simulink model "UAM_Flight_control"  (R2024b)
settings: Solver=FixedStepAuto  StartTime=0.0  StopTime=inf  RelTol=1e-3  EnableMultiTasking=on
undefined symbols (not defined in the file): CityMission, control, controlParams, ControlSampleTime, Cruise_a, DiscIntNeverNeededParam, Earth, FixedWingMission, flightState, FSState, FWControlParams, FWTrimSpeed, HoverMission, params, position, R_WAYPOINTTRANSITION, TransitionMission, uavParam, Vt, w_trim, WGS84, zGround
libraries: slpidlib x56, simulink x32, uavalgslib x7, robotcorelib x2, simulink_extras x2, mspfiltlib x1, aerolibtransform2 x1
(part 12 of 13)

== matlab function UAM_Flight_control/Sensor/Subsystem1/EKF2_Core/EKF2_Algorithm ==
  data: acc input; pos_out output; gyro input; gps_lat input; gps_lon input; gps_alt input; gps_vel input; gps_valid input; baro_alt input; baro_valid input; mag input; mag_valid input; dt input; ref_lat input; ref_lon input; ref_alt input; vel_out output; quat_out output; gyro_bias_out output; accel_bias_out output; wind_vel_out output; terrain_out output; pos_var_out output; vel_var_out output; P_out output; baro_bias_out output; status_out output
function [pos_out, vel_out, quat_out, gyro_bias_out, accel_bias_out, ...
          wind_vel_out, terrain_out, ...
          pos_var_out, vel_var_out, P_out, baro_bias_out, status_out] = ...
    EKF_PX4(acc, gyro, ...
            gps_lat, gps_lon, gps_alt, gps_vel, gps_valid, ...
            baro_alt, baro_valid, ...
            mag, mag_valid, ...
            dt, ref_lat, ref_lon, ref_alt)
%EKF_PX4  PX4 EKF2-equivalent 24-state Extended Kalman Filter (v3.3)
%
%  State vector (24 states):
%    [1:3]   attitude error (rad)      [4:6]   velocity NED (m/s)
%    [7:9]   position NED (m)          [10:12]  gyro bias (rad/s)
%    [13:15] accel bias (m/s^2)        [16:18]  earth mag field (Gauss)
%    [19:21] body mag bias (Gauss)     [22:23]  wind vel NE (m/s)
%    [24]    terrain height (m)
%
%  Update loop (per timestep):
%    1. Buffer sensors  -->  2. Predict state/cov  -->  3. Fuse sensors
%    4. ZUPT / ground damping  -->  5. GSF yaw  -->  6. State resets
%    7. Covariance constraints  -->  8. Output predictor
%
%  Sensors fused:  IMU, GPS (pos/vel/alt), Baro, Magnetometer
%  Not included:   Optical flow, Rangefinder, Airspeed, External vision

% =========================================================================
%  1. TUNING PARAMETERS
% =========================================================================

% --- IMU noise ---
P_GYR_NOISE       = 0.015;       % gyro white noise          (rad/s)
P_ACC_NOISE       = 0.35;        % accel white noise         (m/s^2)
P_GYR_BIAS_NOISE  = 0.001;       % gyro bias random walk     (rad/s^2)
P_ACC_BIAS_NOISE  = 0.01;        % accel bias random walk    (m/s^3)
P_BADACC_PNOISE   = 4.9;         % accel noise during fault  (m/s^2)

% --- Sensor noise ---
P_BARO_NOISE      = 2.0;         % barometer                 (m)
P_GPS_POS_NOISE   = 0.5;         % GPS horizontal position   (m)
P_GPS_VEL_NOISE   = 0.3;         % GPS velocity              (m/s)
P_MAG_NOISE       = 0.05;        % magnetometer body         (Gauss)
P_MAG_BIAS_NOISE  = 0.0001;      % mag body bias drift       (Gauss/s)
P_MAG_EARTH_NOISE = 0.001;       % mag earth field drift     (Gauss/s)
P_HDG_NOISE       = 0.3;         % heading-only mag          (rad)

% --- Environment noise ---
P_WIND_NSD        = 0.1;         % wind velocity             (m/s/sqrt(s))
P_TERR_NOISE      = 5.0;         % terrain height            (m/s)
P_TERR_GRAD       = 0.5;         % terrain gradient          (m/m)

% --- Innovation gates (sigma multiplier) ---
GATE_BARO         = 5.0;
GATE_GPS          = 5.0;
GATE_MAG          = 3.0;
GATE_HDG          = 2.6;

% --- State limits ---
LIM_GYRO_BIAS     = 0.4;         % rad/s
LIM_ACCEL_BIAS    = 0.4;         % m/s^2
LIM_MAG_BIAS      = 0.5;         % Gauss

% --- Bias observability thresholds ---
P_ABL_ACCLIM      = 25.0;        % max accel for bias learn  (m/s^2)
P_ABL_GYRLIM      = 3.0;         % max gyro for bias learn   (rad/s)
P_ABL_TAU         = 0.5;         % maneuver filter tau       (s)
P_IMU_CLIP_THRESH = 39.0;        % IMU clipping threshold    (m/s^2)

% --- Aiding loss fallback ---
P_ZUPT_NOISE      = 0.1;         % zero velocity update      (m/s)
P_ZERO_GYRO_NOISE = 0.01;        % zero gyro update          (rad/s)
P_FAKE_POS_NOISE  = 25.0;        % fake horizontal position  (m)
P_FAKE_HGT_NOISE  = 25.0;        % fake height               (m)

% --- Delay compensation ---
P_GPS_DELAY       = 0.11;        % GPS measurement delay     (s)
BUF_LEN           = 50;          % ring buffer max length

% --- Ground effect ---
P_GND_EFF_DZ      = 4.0;         % propwash deadzone         (m)

% --- EKF-GSF ---
N_GSF             = 5;           % number of GSF models
GSF_RESET_THRESH  = 0.15;        % yaw variance threshold    (rad^2)

% --- Physical constants ---
GRAVITY           = 9.80665;
EARTH_RADIUS      = 6378137.0;
WGS84_E2          = 0.00669437999014;
EARTH_RATE        = 7.2921e-5;    % rad/s

% =========================================================================
%  2. STATE INDICES
% =========================================================================
N_STATES = 24;

IX_ATT = 1:3;       % attitude error
IX_VEL = 4:6;       % velocity NED
IX_POS = 7:9;       % position NED
IX_GB  = 10:12;      % gyro bias
IX_AB  = 13:15;      % accel bias
IX_MI  = 16:18;      % earth magnetic field
IX_MB  = 19:21;      % body magnetic bias
IX_WV  = 22:23;      % wind velocity NE
IX_TR  = 24;         % terrain height

% =========================================================================
%  3. PERSISTENT STATE
% =========================================================================

% --- Core EKF ---
persistent initialized
persistent q_att v_ned p_ned gyro_bias_est accel_bias_est
persistent wind_est terrain_est
persistent P_cov
persistent mag_earth mag_body_bias
persistent baro_bias_est baro_bias_var

% --- Delay ring buffers ---
persistent buf_imu_acc buf_imu_gyro buf_imu_dt
persistent buf_gps_pos buf_gps_vel buf_gps_valid
persistent buf_baro_alt buf_baro_valid
persistent buf_mag_data buf_mag_valid
persistent buf_count delay_steps

% --- Health monitors ---
persistent filt_accel_mag filt_gyro_mag
persistent flag_bad_acc_vert tmr_bad_acc
persistent flag_at_rest tmr_rest
persistent flag_on_ground filt_vibration
persistent lpf_signed_inn tmr_pos_inn tmr_neg_inn
persistent tmr_no_hor_aid tmr_no_ver_aid

% --- Innovation monitors ---
persistent filt_gps_pos_inn filt_gps_vel_inn
persistent tmr_gps_pos_fail tmr_gps_vel_fail
persistent filt_mag_inn tmr_mag_fail

% --- EKF-GSF yaw estimator ---
persistent gsf_yaw gsf_vel gsf_P gsf_weight gsf_converged

% --- Mode flags ---
persistent flag_yaw_aligned flag_mag_3d
persistent cnt_yaw_reset cnt_pos_reset

% --- Output predictor ---
persistent out_q out_v out_p out_initialized

% --- GPS height bias ---
persistent gps_hgt_bias_est gps_hgt_bias_var

% =========================================================================
%  4. INITIALIZATION
% =========================================================================
if isempty(initialized)
    initialized       = false;
    q_att             = [1; 0; 0; 0];
    v_ned             = zeros(3, 1);
    p_ned             = zeros(3, 1);
    gyro_bias_est     = zeros(3, 1);
    accel_bias_est    = zeros(3, 1);
    wind_est          = zeros(2, 1);
    terrain_est       = 0;

    P_cov = diag([ ...
        0.25, 0.25, 0.25, ...       % attitude
        1, 1, 1, ...                 % velocity
        1, 1, 1, ...                 % position
        1e-4, 1e-4, 1e-4, ...       % gyro bias
        0.01, 0.01, 0.01, ...       % accel bias
        0.04, 0.04, 0.04, ...       % mag earth
        0.04, 0.04, 0.04, ...       % mag body
        4, 4, ...                    % wind
        100]);                       % terrain

    mag_earth         = [0.2; 0; 0.4];
    mag_body_bias     = zeros(3, 1);
    baro_bias_est     = 0;
    baro_bias_var     = 1.0;
    gps_hgt_bias_est  = 0;
    gps_hgt_bias_var  = 10.0;

    % Buffers
    buf_imu_acc   = zeros(3, BUF_LEN);
    buf_imu_gyro  = zeros(3, BUF_LEN);
    buf_imu_dt    = zeros(1, BUF_LEN);
    buf_gps_pos   = zeros(3, BUF_LEN);
    buf_gps_vel   = zeros(3, BUF_LEN);
    buf_gps_valid = zeros(1, BUF_LEN);
    buf_baro_alt  = zeros(1, BUF_LEN);
    buf_baro_valid= zeros(1, BUF_LEN);
    buf_mag_data  = zeros(3, BUF_LEN);
    buf_mag_valid = zeros(1, BUF_LEN);
    buf_count     = 0;
    delay_steps   = 0;

    % Monitors
    filt_accel_mag    = GRAVITY;
    filt_gyro_mag     = 0;
    flag_bad_acc_vert = false;
    tmr_bad_acc       = 0;
    flag_at_rest      = true;
    tmr_rest          = 0;
    flag_on_ground    = true;
    filt_vibration    = 0;
    lpf_signed_inn    = 0;
    tmr_pos_inn       = 0;
    tmr_neg_inn       = 0;
    tmr_no_hor_aid    = 0;
    tmr_no_ver_aid    = 0;

    filt_gps_pos_inn  = zeros(2, 1);
    filt_gps_vel_inn  = zeros(3, 1);
    tmr_gps_pos_fail  = 0;
    tmr_gps_vel_fail  = 0;
    filt_mag_inn      = zeros(3, 1);
    tmr_mag_fail      = 0;

    % GSF
    gsf_yaw           = zeros(1, N_GSF);
    gsf_vel           = zeros(2, N_GSF);
    gsf_P             = zeros(3, 3, N_GSF);
    gsf_weight        = ones(1, N_GSF) / N_GSF;
    gsf_converged     = false;

    % Mode
    flag_yaw_aligned  = false;
    flag_mag_3d       = true;
    cnt_yaw_reset     = 0;
    cnt_pos_reset     = 0;

    % Output predictor
    out_q = [1;0;0;0];  out_v = zeros(3,1);  out_p = zeros(3,1);
    out_initialized = false;
end

% =========================================================================
%  5. AUTO-INIT (first valid sensor data)
% =========================================================================
if ~initialized
    delay_steps = min(max(round(P_GPS_DELAY / dt), 1), BUF_LEN);

    % Tilt from accelerometer
    a_norm = acc / max(norm(acc), 1e-6);
    roll0  = atan2(-a_norm(2), -a_norm(3));
    pitch0 = asin(clamp(a_norm(1), -1, 1));

    % Yaw from magnetometer
    yaw0 = 0;
    if mag_valid
        cr = cos(roll0);  sr = sin(roll0);
        cp = cos(pitch0); sp = sin(pitch0);
        mx = mag(1)*cp + mag(2)*sp*sr + mag(3)*sp*cr;
        my = mag(2)*cr - mag(3)*sr;
        yaw0 = atan2(-my, mx);
        flag_yaw_aligned = true;
    end
    q_att = euler2quat(roll0, pitch0, yaw0);

    % Earth magnetic field from first measurement
    if mag_valid
        mag_earth     = quat2dcm(q_att) * mag(:);
        mag_body_bias = zeros(3, 1);
    end

    % Position/velocity from GPS
    if gps_valid
        lat_r = ref_lat * pi / 180;
        p_ned = [(gps_lat - ref_lat) * pi/180 * EARTH_RADIUS;
                 (gps_lon - ref_lon) * pi/180 * EARTH_RADIUS * cos(lat_r);
                 -(gps_alt - ref_alt)];
        v_ned = gps_vel;
    end

    % GSF: spread yaw hypotheses evenly around circle
    for m = 1:N_GSF
        gsf_yaw(m)    = -pi + (m-1) * 2*pi / N_GSF;
        gsf_vel(:, m) = v_ned(1:2);
        gsf_P(:,:,m)  = diag([1, 1, 0.1]);
    end

    out_q = q_att;  out_v = v_ned;  out_p = p_ned;
    initialized = true;
end

% =========================================================================
%  6. SENSOR DELAY BUFFER
% =========================================================================
lat_rad = ref_lat * pi / 180;
gps_ned = [(gps_lat - ref_lat) * pi/180 * EARTH_RADIUS;
           (gps_lon - ref_lon) * pi/180 * EARTH_RADIUS * cos(lat_rad);
           -(gps_alt - ref_alt)];

[d_acc, d_gyro, d_dt, d_gps_ned, d_gps_vel, d_gps_v, ...
 d_baro, d_baro_v, d_mag, d_mag_v] = ...
    push_delay_buffer( ...
        acc, gyro, dt, gps_ned, gps_vel, gps_valid, ...
        baro_alt, baro_valid, mag, mag_valid, ...
        buf_imu_acc, buf_imu_gyro, buf_imu_dt, ...
        buf_gps_pos, buf_gps_vel, buf_gps_valid, ...
        buf_baro_alt, buf_baro_valid, buf_mag_data, buf_mag_valid, ...
        buf_count, delay_steps);

if buf_count < delay_steps
    buf_count = buf_count + 1;
    idx = buf_count;
    buf_imu_acc(:,idx)  = acc;       buf_imu_gyro(:,idx) = gyro;
    buf_imu_dt(idx)     = dt;        buf_gps_pos(:,idx)  = gps_ned;
    buf_gps_vel(:,idx)  = gps_vel;   buf_gps_valid(idx)  = gps_valid;
    buf_baro_alt(idx)   = baro_alt;  buf_baro_valid(idx) = baro_valid;
    buf_mag_data(:,idx) = mag;       buf_mag_valid(idx)  = mag_valid;
else
    % Shift buffers left, push new data to end
    buf_imu_acc  = [buf_imu_acc(:,2:end),  acc];
    buf_imu_gyro = [buf_imu_gyro(:,2:end), gyro];
    buf_imu_dt   = [buf_imu_dt(2:end),     dt];
    buf_gps_pos  = [buf_gps_pos(:,2:end),  gps_ned];
    buf_gps_vel  = [buf_gps_vel(:,2:end),  gps_vel];
    buf_gps_valid= [buf_gps_valid(2:end),  gps_valid];
    buf_baro_alt = [buf_baro_alt(2:end),   baro_alt];
    buf_baro_valid=[buf_baro_valid(2:end),  baro_valid];
    buf_mag_data = [buf_mag_data(:,2:end), mag];
    buf_mag_valid= [buf_mag_valid(2:end),  mag_valid];
end

% =========================================================================
%  7. IMU PREPROCESSING
% =========================================================================
gyro_corrected = d_gyro - gyro_bias_est;
acc_corrected  = d_acc  - accel_bias_est;
imu_clipping   = abs(d_acc) > P_IMU_CLIP_THRESH;

% Filtered maneuver level
alpha_filt = clamp(d_dt / P_ABL_TAU, 0, 1);
filt_accel_mag = max(norm(acc_corrected), (1 - alpha_filt) * filt_accel_mag);
filt_gyro_mag  = max(norm(gyro_corrected),(1 - alpha_filt) * filt_gyro_mag);
is_high_maneuver = (filt_gyro_mag > P_ABL_GYRLIM) || ...
                   (filt_accel_mag > P_ABL_ACCLIM);

% =========================================================================
%  8. FAULT DETECTION
% =========================================================================

% --- Bad vertical accelerometer ---
vert_accel_err = abs(acc_corrected(3) + GRAVITY);
if vert_accel_err > 2.0
    tmr_bad_acc = tmr_bad_acc + d_dt;
    if tmr_bad_acc > 1.0, flag_bad_acc_vert = true; end
else
    tmr_bad_acc = max(tmr_bad_acc - d_dt, 0);
    if tmr_bad_acc < 0.5, flag_bad_acc_vert = false; end
end

% --- Vehicle at rest (requires no vibration) ---
is_gyro_still  = norm(gyro_corrected) < 0.05;
is_accel_still = abs(norm(acc_corrected) - GRAVITY) < 0.5;
is_vel_low     = norm(v_ned) < 0.1;
if is_gyro_still && is_accel_still && is_vel_low
    tmr_rest = tmr_rest + d_dt;
    if tmr_rest > 1.0, flag_at_rest = true; end
else
    tmr_rest = 0;
    flag_at_rest = false;
end

% --- On-ground (works even with motor vibration) ---
is_alt_low = -p_ned(3) < 2.0;
is_vz_low  = abs(v_ned(3)) < 0.5;
flag_on_ground = is_alt_low && (norm(v_ned) < 1.0) && is_vz_low;

% --- Motor vibration detection (proxy for motors active) ---
vib_alpha = clamp(d_dt / 0.5, 0, 1);
filt_vibration = (1 - vib_alpha) * filt_vibration + ...
                  vib_alpha * abs(norm(d_acc) - GRAVITY);
flag_motor_vibration = (filt_vibration > 0.5) && (filt_vibration < 15.0);
flag_gnd_effect = flag_on_ground || (is_alt_low && flag_motor_vibration);

% =========================================================================
%  9. STATE PREDICTION
% =========================================================================

% --- Attitude (exponential map quaternion integration) ---
R_body2ned = quat2dcm(q_att);
earth_rate_NED  = [EARTH_RATE*cos(lat_rad); 0; -EARTH_RATE*sin(lat_rad)];
earth_rate_body = R_body2ned' * earth_rate_NED;

delta_angle = (gyro_corrected - earth_rate_body) * d_dt;
q_pred = qmult(q_att, expmap_quat(delta_angle));
q_pred = q_pred / norm(q_pred);

% --- Velocity (NED frame with Coriolis + transport rate) ---
R_pred = quat2dcm(q_pred);
acc_ned = R_pred * acc_corrected;
coriolis = -2 * cross3(earth_rate_NED, v_ned);

% WGS84 ellipsoid radii of curvature
sin_lat = sin(lat_rad);
den_lat = sqrt(1 - WGS84_E2 * sin_lat^2);
r_meridian = EARTH_RADIUS * (1 - WGS84_E2) / (den_lat^3);
r_prime    = EARTH_RADIUS / den_lat;
altitude   = -p_ned(3);

omega_transport = [ v_ned(2) / (r_prime + altitude);
                   -v_ned(1) / (r_meridian + altitude);
                   -v_ned(2) * tan(lat_rad) / (r_prime + altitude)];
transport = -cross3(omega_transport, v_ned);

v_pred = v_ned + (acc_ned + [0;0;GRAVITY] + coriolis + transport) * d_dt;

% --- Position (trapezoidal integration) ---
p_pred = p_ned + (v_ned + v_pred) * 0.5 * d_dt;

% =========================================================================
%  10. COVARIANCE PREDICTION
% =========================================================================

% State transition Jacobian (first-order)
F = eye(N_STATES);
F(IX_ATT, IX_GB)  = -eye(3) * d_dt;
F(IX_VEL, IX_ATT) = -R_pred * skew3(acc_corrected) * d_dt;
F(IX_VEL, IX_AB)  = -R_pred * d_dt;
F(IX_POS, IX_VEL) =  eye(3) * d_dt;

% Process noise
Q = zeros(N_STATES);
Q(IX_ATT, IX_ATT) = eye(3) * (P_GYR_NOISE * d_dt)^2;
Q(IX_VEL, IX_VEL) = eye(3) * (P_ACC_NOISE * d_dt)^2;

P_pred = F * P_cov * F' + Q;

% Bias process noise (conditional for accel bias)
accel_var = P_ACC_NOISE^2 * ones(3, 1);
if flag_bad_acc_vert || any(imu_clipping)
    accel_var = P_BADACC_PNOISE^2 * ones(3, 1);
end
for i = 1:3
    P_pred(IX_GB(i), IX_GB(i)) = P_pred(IX_GB(i), IX_GB(i)) + ...
                                  (P_GYR_BIAS_NOISE * d_dt)^2;
    if P_pred(IX_AB(i), IX_AB(i)) < accel_var(i)
        P_pred(IX_AB(i), IX_AB(i)) = P_pred(IX_AB(i), IX_AB(i)) + ...
                                      (P_ACC_BIAS_NOISE * d_dt)^2;
    end
end
for i = IX_MI, P_pred(i,i) = P_pred(i,i) + (P_MAG_EARTH_NOISE*d_dt)^2; end
for i = IX_MB, P_pred(i,i) = P_pred(i,i) + (P_MAG_BIAS_NOISE*d_dt)^2;  end
for i = IX_WV, P_pred(i,i) = P_pred(i,i) + (P_WIND_NSD*d_dt)^2;        end

terr_pn = (P_TERR_NOISE*d_dt)^2 + ...
          (P_TERR_GRAD*d_dt)^2 * (v_pred(1)^2 + v_pred(2)^2);
P_pred(IX_TR, IX_TR) = P_pred(IX_TR, IX_TR) + terr_pn;
P_pred = 0.5 * (P_pred + P_pred');

% =========================================================================
%  11. BIAS INHIBIT
% =========================================================================
gb_inhibit = false(3, 1);
ab_inhibit = false(3, 1);
for i = 1:3
    if abs(gyro_corrected(i)) > 5.0
        gb_inhibit(i) = true;
    end
end
inhibit_all_ab = is_high_maneuver || flag_bad_acc_vert;
for i = 1:3
    ab_inhibit(i) = inhibit_all_ab || imu_clipping(i);
    if ~flag_at_rest && abs(R_pred(3,i)) < sin(15*pi/180)
        ab_inhibit(i) = true;        % not observable
    end
end

% =========================================================================
%  12. MEASUREMENT UPDATES (sequential scalar fusion)
% =========================================================================
q_u  = q_pred;     v_u  = v_pred;    p_u  = p_pred;
gb_u = gyro_bias_est;  ab_u = accel_bias_est;
wv_u = wind_est;   tr_u = terrain_est;
P_u  = P_pred;

did_fuse_gps = false;
did_fuse_hgt = false;
mag_hdg_ratio = 0;

% Shorthand for repeated fusion call arguments
FARGS = {IX_ATT, IX_VEL, IX_POS, IX_GB, IX_AB, ...
         IX_MI, IX_MB, IX_WV, IX_TR, ...
         LIM_GYRO_BIAS, LIM_ACCEL_BIAS, LIM_MAG_BIAS};

% ----- 12a. BAROMETER HEIGHT (primary reference) -----------------------
if d_baro_v
    H_b = zeros(1, N_STATES);  H_b(9) = 1;
    obs_baro = -(d_baro - ref_alt) - baro_bias_est;
    inn_b = obs_baro - p_u(3);

    % One-sided deadzone: suppress only negative innovations (propwash)
    %   inn_b < 0 means baro reads higher than EKF (low pressure from propwash)
    %   If |inn_b| < DZ  → zero out (inside deadzone)
    %   If |inn_b| >= DZ → shift by DZ toward zero
    R_baro = P_BARO_NOISE;
    if flag_gnd_effect && P_GND_EFF_DZ > 0
        if inn_b < 0
            if inn_b > -P_GND_EFF_DZ
                inn_b = 0;                    % inside deadzone
            else
                inn_b = inn_b + P_GND_EFF_DZ; % shift toward zero
            end
        end
        if flag_motor_vibration
            R_baro = P_BARO_NOISE * 3.0;
        end
    end

    S_b = H_b * P_u * H_b' + R_baro^2;
    test_ratio = inn_b^2 / (GATE_BARO^2 * S_b);

    % Clamp during bad vertical accel (don't reject, just limit)
    if flag_bad_acc_vert && test_ratio >= 1.0
        inn_b = clamp(inn_b, -GATE_BARO*sqrt(S_b), GATE_BARO*sqrt(S_b));
        test_ratio = 0.99;
    end

    if test_ratio < 1.0
        K_b = P_u * H_b' / S_b;
        K_b = apply_inhibit(K_b, gb_inhibit, ab_inhibit, IX_GB, IX_AB);
        [q_u,v_u,p_u,gb_u,ab_u,mag_earth,mag_body_bias,wv_u,tr_u] = ...
            fuse_state(q_u,v_u,p_u,gb_u,ab_u,mag_earth,mag_body_bias, ...
                       wv_u,tr_u, K_b, inn_b, FARGS{:});
        P_u = joseph_update(P_u, K_b, H_b, R_baro^2, N_STATES);
        did_fuse_hgt = true;
        tmr_no_ver_aid = 0;
    end
end

% ----- 12b. BARO BIAS ESTIMATOR ----------------------------------------
BIAS_MON_TIME = 10.0;
baro_bias_pn = 0.01^2 * d_dt;
if abs(lpf_signed_inn) > 0.2 || tmr_pos_inn > BIAS_MON_TIME || ...
   tmr_neg_inn > BIAS_MON_TIME
    baro_bias_pn = baro_bias_pn * 10.0;
end
if flag_gnd_effect && flag_motor_vibration
    baro_bias_pn = baro_bias_pn * 50.0;  % fast tracking during propwash
end
baro_bias_var = clamp(baro_bias_var + baro_bias_pn, 1e-8, 100);

if d_baro_v
    bi = (-(d_baro - ref_alt) + p_u(3)) - baro_bias_est;
    Si = baro_bias_var + P_BARO_NOISE^2 + P_u(9,9);
    tr_bi = bi^2 / (25 * Si);
    if tr_bi < 1.0
        Kb = baro_bias_var / Si;
        baro_bias_est = baro_bias_est + Kb * bi;
        baro_bias_var = (1 - Kb) * baro_bias_var;
    end
    lpf_a = clamp(d_dt / BIAS_MON_TIME, 0, 1);
    lpf_signed_inn = (1-lpf_a)*lpf_signed_inn + lpf_a*sign(bi)*min(tr_bi,1);
    if bi > 0
        tmr_pos_inn = 0;  tmr_neg_inn = tmr_neg_inn + d_dt;
    else
        tmr_neg_inn = 0;  tmr_pos_inn = tmr_pos_inn + d_dt;
    end
end

% ----- 12c. GPS HORIZONTAL POSITION ------------------------------------
gps_pos_rejected = false;
if d_gps_v
    rej_cnt = 0;
    for ax = 1:2
        H = zeros(1,N_STATES);  H(6+ax) = 1;
        inn = d_gps_ned(ax) - p_u(ax);
        S = H*P_u*H' + P_GPS_POS_NOISE^2;
        tr = inn^2 / (GATE_GPS^2 * S);

        af = clamp(d_dt / 0.5, 0, 1);
        filt_gps_pos_inn(ax) = (1-af)*filt_gps_pos_inn(ax) + ...
                                af*sign(inn)*min(tr, 1);
        if tr < 1.0
            K = apply_inhibit(P_u*H'/S, gb_inhibit, ab_inhibit, IX_GB, IX_AB);
            [q_u,v_u,p_u,gb_u,ab_u,mag_earth,mag_body_bias,wv_u,tr_u] = ...
                fuse_state(q_u,v_u,p_u,gb_u,ab_u,mag_earth,mag_body_bias,...
                           wv_u,tr_u, K, inn, FARGS{:});
            P_u = joseph_update(P_u, K, H, P_GPS_POS_NOISE^2, N_STATES);
            did_fuse_gps = true;
            tmr_no_hor_aid = 0;
        else
            rej_cnt = rej_cnt + 1;
        end
    end
    gps_pos_rejected = (rej_cnt == 2);
end
tmr_gps_pos_fail = update_fail_timer(tmr_gps_pos_fail, ...
                    gps_pos_rejected || ~d_gps_v, d_dt);

% ----- 12d. GPS VELOCITY -----------------------------------------------
gps_vel_rejected = false;
if d_gps_v
    rej_cnt = 0;
    for ax = 1:3
        H = zeros(1,N_STATES);  H(3+ax) = 1;
        inn = d_gps_vel(ax) - v_u(ax);
        R_v = P_GPS_VEL_NOISE^2;
        if ax == 3, R_v = (1.5 * P_GPS_VEL_NOISE)^2; end  % vz: 1.5x noise
        S = H*P_u*H' + R_v;
        tr = inn^2 / (GATE_GPS^2 * S);

        af = clamp(d_dt / 0.5, 0, 1);
        filt_gps_vel_inn(ax) = (1-af)*filt_gps_vel_inn(ax) + ...
                                af*sign(inn)*min(tr, 1);
        if tr < 1.0
            K = apply_inhibit(P_u*H'/S, gb_inhibit, ab_inhibit, IX_GB, IX_AB);
            [q_u,v_u,p_u,gb_u,ab_u,mag_earth,mag_body_bias,wv_u,tr_u] = ...
                fuse_state(q_u,v_u,p_u,gb_u,ab_u,mag_earth,mag_body_bias,...
                           wv_u,tr_u, K, inn, FARGS{:});
            P_u = joseph_update(P_u, K, H, R_v, N_STATES);
            did_fuse_gps = true;
        else
            rej_cnt = rej_cnt + 1;
        end
    end
    gps_vel_rejected = (rej_cnt == 3);
end
tmr_gps_vel_fail = update_fail_timer(tmr_gps_vel_fail, ...
                    gps_vel_rejected || ~d_gps_v, d_dt);

% ----- 12e. GPS ALTITUDE (with bias estimator) -------------------------
gps_hgt_bias_var = min(gps_hgt_bias_var + 0.02^2 * d_dt, 100);
if d_gps_v
    H = zeros(1,N_STATES);  H(9) = 1;
    R_ga = (1.5 * P_GPS_POS_NOISE)^2;
    obs_gps_z = d_gps_ned(3) - gps_hgt_bias_est;
    inn = obs_gps_z - p_u(3);
    S = H*P_u*H' + R_ga + gps_hgt_bias_var;

    if flag_bad_acc_vert
        inn = clamp(inn, -GATE_GPS*sqrt(S), GATE_GPS*sqrt(S));
    end
    if inn^2 < GATE_GPS^2 * S
        K = apply_inhibit(P_u*H'/S, gb_inhibit, ab_inhibit, IX_GB, IX_AB);
        [q_u,v_u,p_u,gb_u,ab_u,mag_earth,mag_body_bias,wv_u,tr_u] = ...
            fuse_state(q_u,v_u,p_u,gb_u,ab_u,mag_earth,mag_body_bias,...
                       wv_u,tr_u, K, inn, FARGS{:});
        P_u = joseph_update(P_u, K, H, R_ga + gps_hgt_bias_var, N_STATES);
        did_fuse_hgt = true;
        tmr_no_ver_aid = 0;
    end

    % Bias estimator update
    gi = d_gps_ned(3) - p_u(3) - gps_hgt_bias_est;
    Si_g = gps_hgt_bias_var + R_ga + P_u(9,9);
    if gi^2 < 25*Si_g && Si_g > 1e-6
        Kg = gps_hgt_bias_var / Si_g;
        gps_hgt_bias_est = gps_hgt_bias_est + Kg * gi;
        gps_hgt_bias_var = (1 - Kg) * gps_hgt_bias_var;
    end
end

% ----- 12f. MAGNETOMETER -----------------------------------------------
R_dcm = quat2dcm(q_u);
R_dcm_t = R_dcm';
pitch_now = asin(clamp(-R_dcm(1,3), -1, 1));

% Mode selection: 3D or heading-only
mag_disturbed = false;
if d_mag_v
    if abs(norm(d_mag) - norm(mag_earth)) > 0.3 * norm(mag_earth)
        mag_disturbed = true;
    end
end
if abs(pitch_now) > 60*pi/180 || tmr_mag_fail > 3.0 || mag_disturbed
    flag_mag_3d = false;
else
    flag_mag_3d = true;
end

if d_mag_v
    if flag_mag_3d
        % --- 3D magnetometer fusion ---
        mag_pred = R_dcm_t * mag_earth + mag_body_bias;
        allow_tilt = abs(pitch_now) < 45*pi/180;
        mag_rej = 0;

        for ax = 1:3
            dMdA = -R_dcm_t * skew3(mag_earth);
            H = zeros(1,N_STATES);
            H(IX_ATT) = dMdA(ax,:);
            H(IX_MI)  = R_dcm_t(ax,:);
            H(IX_MB(ax)) = 1;

            inn = d_mag(ax) - mag_pred(ax);
            S = H*P_u*H' + P_MAG_NOISE^2;
            tr = inn^2 / (GATE_MAG^2 * S);

            af = clamp(d_dt / 0.5, 0, 1);
            filt_mag_inn(ax) = (1-af)*filt_mag_inn(ax) + af*sign(inn)*min(tr,1);

            if tr < 1.0 && S > 0
                K = apply_inhibit(P_u*H'/S, gb_inhibit, ab_inhibit, IX_GB, IX_AB);
                if ~allow_tilt
                    K(1) = 0;  K(2) = 0;
                    K(IX_GB(1)) = 0;  K(IX_GB(2)) = 0;
                end
                [q_u,v_u,p_u,gb_u,ab_u,mag_earth,mag_body_bias,wv_u,tr_u]=...
                    fuse_state(q_u,v_u,p_u,gb_u,ab_u,mag_earth,...
                               mag_body_bias,wv_u,tr_u,K,inn,FARGS{:});
                P_u = joseph_update(P_u, K, H, P_MAG_NOISE^2, N_STATES);

                R_dcm = quat2dcm(q_u);  R_dcm_t = R_dcm';
                mag_pred = R_dcm_t * mag_earth + mag_body_bias;
            else
                mag_rej = mag_rej + 1;
            end
        end
        tmr_mag_fail = update_fail_timer(tmr_mag_fail, mag_rej==3, d_dt);

    else
        % --- Heading-only magnetometer fusion ---
        mag_NED = R_dcm * d_mag;
        Bx = mag_NED(1);  By = mag_NED(2);
        D_meas = Bx^2 + By^2;
        D_pred = mag_earth(1)^2 + mag_earth(2)^2;

        if D_meas > 0.01 && D_pred > 0.01
            inn = wrapToPi(atan2(By, Bx) - atan2(mag_earth(2), mag_earth(1)));

            H = zeros(1, N_STATES);
            H(3) = -1;                                 % yaw only
            H(IX_MI(1)) =  mag_earth(2) / D_pred;
            H(IX_MI(2)) = -mag_earth(1) / D_pred;

            S = H*P_u*H' + P_HDG_NOISE^2;
            tr = inn^2 / (GATE_HDG^2 * S);
            mag_hdg_ratio = tr;

            if tr < 1.0 && S > 0
                K = apply_inhibit(P_u*H'/S, gb_inhibit, ab_inhibit, IX_GB, IX_AB);
                K(1) = 0;  K(2) = 0;
                K(IX_GB(1)) = 0;  K(IX_GB(2)) = 0;
                [q_u,v_u,p_u,gb_u,ab_u,mag_earth,mag_body_bias,wv_u,tr_u]=...
                    fuse_state(q_u,v_u,p_u,gb_u,ab_u,mag_earth,...
                               mag_body_bias,wv_u,tr_u,K,inn,FARGS{:});
                P_u = joseph_update(P_u, K, H, P_HDG_NOISE^2, N_STATES);
                tmr_mag_fail = max(tmr_mag_fail - d_dt, 0);
            else
                tmr_mag_fail = tmr_mag_fail + d_dt;
            end
        end
    end
end

% ----- 12g. GRAVITY VECTOR FUSION --------------------------------------
if ~is_high_maneuver && ~flag_bad_acc_vert
    acc_mag = norm(acc_corrected);
    if acc_mag > 0.5*GRAVITY && acc_mag < 1.5*GRAVITY
        R_g = quat2dcm(q_u);
        grav_pred = R_g' * [0;0;GRAVITY];
        grav_meas = acc_corrected / acc_mag * GRAVITY;
        R_grav = 1.0;

        for ax = 1:2
            dGdA = -R_g' * skew3([0;0;GRAVITY]);
            H_g = zeros(1, N_STATES);
            H_g(IX_ATT) = dGdA(ax,:);
            H_g(IX_AB(ax)) = -1;

            inn_g = grav_meas(ax) - grav_pred(ax);
            S_g = H_g*P_u*H_g' + R_grav;
            if inn_g^2 < 9*S_g && S_g > 0
                K_g = apply_inhibit(P_u*H_g'/S_g, gb_inhibit, ab_inhibit, IX_GB, IX_AB);
                K_g(3) = 0;  K_g(IX_GB(3)) = 0;    % no yaw from gravity
                [q_u,v_u,p_u,gb_u,ab_u,mag_earth,mag_body_bias,wv_u,tr_u]=...
                    fuse_state(q_u,v_u,p_u,gb_u,ab_u,mag_earth,...
                               mag_body_bias,wv_u,tr_u,K_g,inn_g,FARGS{:});
                P_u = joseph_update(P_u, K_g, H_g, R_grav, N_STATES);
            end
        end
    end
end

% =========================================================================
%  13. VELOCITY CONSTRAINTS
% =========================================================================

% --- ZUPT (vehicle at rest) ---
if flag_at_rest
    for ax = 1:3
        H = zeros(1,N_STATES);  H(3+ax) = 1;
        inn = -v_u(ax);
        S = H*P_u*H' + P_ZUPT_NOISE^2;
        if inn^2 < 25*S
            K = apply_inhibit(P_u*H'/S, gb_inhibit, ab_inhibit, IX_GB, IX_AB);
            [q_u,v_u,p_u,gb_u,ab_u,mag_earth,mag_body_bias,wv_u,tr_u]=...
                fuse_state(q_u,v_u,p_u,gb_u,ab_u,mag_earth,...
                           mag_body_bias,wv_u,tr_u,K,inn,FARGS{:});
            P_u = joseph_update(P_u, K, H, P_ZUPT_NOISE^2, N_STATES);
        end
    end
end

% --- On-ground velocity damping (motors running but not flying) ---
if flag_on_ground && ~flag_at_rest
    % Vertical velocity → zero (tight)
    H = zeros(1,N_STATES);  H(6) = 1;
    inn_vz = -v_u(3);
    R_vz = 0.5^2;
    S_vz = H*P_u*H' + R_vz;
    if inn_vz^2 < 25*S_vz
        K = apply_inhibit(P_u*H'/S_vz, gb_inhibit, ab_inhibit, IX_GB, IX_AB);
        [q_u,v_u,p_u,gb_u,ab_u,mag_earth,mag_body_bias,wv_u,tr_u]=...
            fuse_state(q_u,v_u,p_u,gb_u,ab_u,mag_earth,...
                       mag_body_bias,wv_u,tr_u,K,inn_vz,FARGS{:});
        P_u = joseph_update(P_u, K, H, R_vz, N_STATES);
    end

    % Horizontal velocity → zero (looser)
    R_vh = 2.0^2;
    for ax = 1:2
        H = zeros(1,N_STATES);  H(3+ax) = 1;
        inn_vh = -v_u(ax);
        S_vh = H*P_u*H' + R_vh;
        if inn_vh^2 < 25*S_vh
            K = apply_inhibit(P_u*H'/S_vh, gb_inhibit, ab_inhibit, IX_GB, IX_AB);
            [q_u,v_u,p_u,gb_u,ab_u,mag_earth,mag_body_bias,wv_u,tr_u]=...
                fuse_state(q_u,v_u,p_u,gb_u,ab_u,mag_earth,...
                           mag_body_bias,wv_u,tr_u,K,inn_vh,FARGS{:});
            P_u = joseph_update(P_u, K, H, R_vh, N_STATES);
        end
    end
end

% --- Zero gyro update (at rest only) ---
if flag_at_rest
    for ax = 1:3
        H = zeros(1,N_STATES);  H(IX_GB(ax)) = -1;
        inn = -(d_gyro(ax) - gb_u(ax));
        S = H*P_u*H' + P_ZERO_GYRO_NOISE^2;
        if S > 0 && inn^2 < 25*S
            K = P_u*H'/S;
            [q_u,v_u,p_u,gb_u,ab_u,mag_earth,mag_body_bias,wv_u,tr_u]=...
                fuse_state(q_u,v_u,p_u,gb_u,ab_u,mag_earth,...
                           mag_body_bias,wv_u,tr_u,K,inn,FARGS{:});
            P_u = joseph_update(P_u, K, H, P_ZERO_GYRO_NOISE^2, N_STATES);
        end
    end
end

% --- Fake position / height aiding ---
if ~did_fuse_gps, tmr_no_hor_aid = tmr_no_hor_aid + d_dt; end
if ~did_fuse_hgt, tmr_no_ver_aid = tmr_no_ver_aid + d_dt; end

if tmr_no_hor_aid > 5.0
    for ax = 1:2
        H = zeros(1,N_STATES);  H(6+ax) = 1;
        S = H*P_u*H' + P_FAKE_POS_NOISE^2;
        P_u = joseph_update(P_u, P_u*H'/S, H, P_FAKE_POS_NOISE^2, N_STATES);
    end
end
if tmr_no_ver_aid > 5.0
    H = zeros(1,N_STATES);  H(9) = 1;
    S = H*P_u*H' + P_FAKE_HGT_NOISE^2;
    P_u = joseph_update(P_u, P_u*H'/S, H, P_FAKE_HGT_NOISE^2, N_STATES);
end

% =========================================================================
%  14. EKF-GSF YAW ESTIMATOR
% =========================================================================
[roll_now, pitch_now_e, yaw_now] = quat2euler(q_u);

% Predict all models
for m = 1:N_GSF
    sr = sin(roll_now);  cr = cos(roll_now);  cp = cos(pitch_now_e);
    yaw_rate = gyro_corrected(3);
    if abs(cp) > 1e-6
        yaw_rate = gyro_corrected(2)*sr/cp + gyro_corrected(3)*cr/cp;
    end
    gsf_yaw(m) = wrapToPi(gsf_yaw(m) + yaw_rate * d_dt);

    R_gsf = euler2dcm(roll_now, pitch_now_e, gsf_yaw(m));
    a_ned = R_gsf * acc_corrected;
    gsf_vel(:,m) = gsf_vel(:,m) + a_ned(1:2) * d_dt;

    cy = cos(gsf_yaw(m));  sy = sin(gsf_yaw(m));
    dv_dpsi = [(-acc_corrected(1)*sy - acc_corrected(2)*cy) * d_dt;
               ( acc_corrected(1)*cy - acc_corrected(2)*sy) * d_dt];
    Fm = eye(3);  Fm(1,3) = dv_dpsi(1);  Fm(2,3) = dv_dpsi(2);
    Qm = diag([(P_ACC_NOISE*d_dt)^2, (P_ACC_NOISE*d_dt)^2, (P_GYR_NOISE*d_dt)^2]);
    gsf_P(:,:,m) = Fm * gsf_P(:,:,m) * Fm' + Qm;
end

% Update with GPS velocity
if d_gps_v && did_fuse_gps
    for m = 1:N_GSF
        inn_g = d_gps_vel(1:2) - gsf_vel(:,m);
        cy = cos(gsf_yaw(m));  sy = sin(gsf_yaw(m));
        dv = [(-acc_corrected(1)*sy - acc_corrected(2)*cy)*d_dt;
              ( acc_corrected(1)*cy - acc_corrected(2)*sy)*d_dt];
        Hm = [1,0,dv(1); 0,1,dv(2)];
        Rm = P_GPS_VEL_NOISE^2 * eye(2);
        Sm = Hm * gsf_P(:,:,m) * Hm' + Rm;

        det_S = Sm(1,1)*Sm(2,2) - Sm(1,2)*Sm(2,1);
        if det_S > 1e-6
            Si = [Sm(2,2),-Sm(1,2); -Sm(2,1),Sm(1,1)] / det_S;

            nis = inn_g' * Si * inn_g;
            if nis > 25, inn_g = inn_g * sqrt(25/nis); nis = 25; end

            Km = gsf_P(:,:,m) * Hm' * Si;
            dx = Km * inn_g;
            gsf_vel(:,m) = gsf_vel(:,m) + dx(1:2);
            gsf_yaw(m) = wrapToPi(gsf_yaw(m) + dx(3));
            gsf_P(:,:,m) = (eye(3) - Km*Hm) * gsf_P(:,:,m);

            gsf_weight(m) = gsf_weight(m) * exp(-0.5*nis) / sqrt(abs(det_S));
        end
    end
    wt_sum = sum(gsf_weight);
    if wt_sum > 1e-30
        gsf_weight = gsf_weight / wt_sum;
    else
        gsf_weight = ones(1,N_GSF) / N_GSF;
    end
end

% Composite estimate
s_sum = sum(gsf_weight .* sin(gsf_yaw));
c_sum = sum(gsf_weight .* cos(gsf_yaw));
gsf_yaw_est = atan2(s_sum, c_sum);

% Mixture variance
gsf_yaw_var = 0;
for m = 1:N_GSF
    d_yaw = wrapToPi(gsf_yaw(m) - gsf_yaw_est);
    gsf_yaw_var = gsf_yaw_var + gsf_weight(m) * (gsf_P(3,3,m) + d_yaw^2);
end
gsf_yaw_var = max(gsf_yaw_var, 1e-4);
gsf_converged = gsf_yaw_var < GSF_RESET_THRESH;

% =========================================================================
%  15. STATE RESETS
% =========================================================================

% --- Yaw reset from GSF ---
yaw_failing = tmr_mag_fail > 5.0 || mag_hdg_ratio > 1.0;
if gsf_converged && (~flag_yaw_aligned || (yaw_failing && ~flag_at_rest))
    dq = euler2quat(0, 0, wrapToPi(gsf_yaw_est - yaw_now));
    q_u = qmult(dq, q_u);
    q_u = q_u / norm(q_u);
    P_u(3,:) = 0;  P_u(:,3) = 0;
    P_u(3,3) = max(gsf_yaw_var, 1e-4);
    flag_yaw_aligned = true;
    cnt_yaw_reset = cnt_yaw_reset + 1;
    tmr_mag_fail = 0;
end

% --- Position reset from GPS ---
if tmr_gps_pos_fail > 5.0 && d_gps_v && ~gps_pos_rejected
    p_u(1:2) = d_gps_ned(1:2);
    P_u(7,:)=0; P_u(:,7)=0; P_u(8,:)=0; P_u(:,8)=0;
    P_u(7,7) = P_GPS_POS_NOISE^2;
    P_u(8,8) = P_GPS_POS_NOISE^2;
    tmr_gps_pos_fail = 0;
    cnt_pos_reset = cnt_pos_reset + 1;
end

% --- Velocity reset from GPS ---
if tmr_gps_vel_fail > 5.0 && d_gps_v && ~gps_vel_rejected
    v_u = d_gps_vel;
    for ax = 4:6
        P_u(ax,:)=0; P_u(:,ax)=0;
    end
    P_u(4,4)=P_GPS_VEL_NOISE^2; P_u(5,5)=P_GPS_VEL_NOISE^2;
    P_u(6,6)=P_GPS_VEL_NOISE^2;
    tmr_gps_vel_fail = 0;
end

% =========================================================================
%  16. COVARIANCE HEALTH
% =========================================================================
cov_max = [1,1,1, 1e6,1e6,1e6, 1e6,1e6,1e6, .1,.1,.1, .1,.1,.1, ...
           1,1,1, 1,1,1, 1e6,1e6, 1e4];
cov_min = [1e-9,1e-9,1e-9, 1e-6,1e-6,1e-6, 1e-6,1e-6,1e-6, ...
           1e-9,1e-9,1e-9, 1e-9,1e-9,1e-9, 1e-6,1e-6,1e-6, ...
           1e-6,1e-6,1e-6, 1e-6,1e-6, 0];

for i = 1:N_STATES
    if P_u(i,i) < cov_min(i)
        P_u(i,i) = cov_min(i);
    elseif P_u(i,i) > cov_max(i)
        % Fuse zero-innovation to reduce ~10% (preserves cross-correlation)
        R_s = 10 * P_u(i,i);
        Hs = zeros(1,N_STATES);  Hs(i) = 1;
        P_u = joseph_update(P_u, P_u*Hs'/(P_u(i,i)+R_s), Hs, R_s, N_STATES);
    end
end
P_u = 0.5 * (P_u + P_u');

% =========================================================================
%  17. STORE DELAYED STATE
% =========================================================================
q_att         = q_u;
v_ned         = v_u;
p_ned         = p_u;
gyro_bias_est = gb_u;
accel_bias_est= ab_u;
wind_est      = wv_u;
terrain_est   = tr_u;
P_cov         = P_u;

% =========================================================================
%  18. OUTPUT PREDICTOR (replay IMU from delayed → current time)
% =========================================================================
oq = q_u;  ov = v_u;  op = p_u;

if buf_count >= delay_steps && delay_steps > 0
    for k = 1:delay_steps
        gk = buf_imu_gyro(:,k) - gb_u;
        ak = buf_imu_acc(:,k)  - ab_u;
        dtk = buf_imu_dt(k);

        Rk = quat2dcm(oq);
        d_ang = (gk - Rk' * earth_rate_NED) * dtk;
        oq = qmult(oq, expmap_quat(d_ang));
        oq = oq / norm(oq);

        a_ned_k = quat2dcm(oq) * ak;
        ov = ov + (a_ned_k + [0;0;GRAVITY]) * dtk;
        op = op + ov * dtk;
    end
end

% Smooth transition (prevent output jumps)
TAU_SMOOTH = 0.15;
alpha_s = clamp(dt / (dt + TAU_SMOOTH), 0, 1);

if out_initialized
    out_v = out_v + alpha_s * (ov - out_v);
    out_p = out_p + alpha_s * (op - out_p);

    q_err = qmult(qconj(out_q), oq);
    if q_err(1) < 0, q_err = -q_err; end
    att_corr = alpha_s * 2 * q_err(2:4);
    out_q = qmult(expmap_quat(att_corr), out_q);
    out_q = out_q / norm(out_q);
else
    out_q = oq;  out_v = ov;  out_p = op;
    out_initialized = true;
end

% =========================================================================
%  19. OUTPUTS
% =========================================================================
status_out = [ ...
    double(flag_at_rest);        %  1: vehicle at rest
    double(flag_bad_acc_vert);   %  2: bad vertical accel
    double(tmr_no_hor_aid>10);   %  3: horizontal dead reckoning
    double(tmr_no_ver_aid>10);   %  4: vertical dead reckoning
    double(did_fuse_gps);        %  5: GPS fused this step
    double(did_fuse_hgt);        %  6: height fused this step
    double(flag_yaw_aligned);    %  7: yaw is aligned
    double(gsf_converged);       %  8: GSF yaw converged
    double(flag_mag_3d);         %  9: using 3D mag fusion
    double(cnt_yaw_reset)];      % 10: yaw reset count

quat_out       = out_q;
vel_out        = out_v;
pos_out        = out_p;
gyro_bias_out  = gb_u;
accel_bias_out = ab_u;
wind_vel_out   = wv_u;
terrain_out    = tr_u;
baro_bias_out  = baro_bias_est;
P_out          = P_u;
pos_var_out    = [P_u(7,7); P_u(8,8); P_u(9,9)];
vel_var_out    = [P_u(4,4); P_u(5,5); P_u(6,6)];
end


% #########################################################################
%  HELPER FUNCTIONS
% #########################################################################

% ---- Clamp value to [lo, hi] -------------------------------------------
function y = clamp(x, lo, hi)
    y = min(max(x, lo), hi);
end

% ---- Skew-symmetric matrix ---------------------------------------------
function S = skew3(v)
    S = [0,-v(3),v(2); v(3),0,-v(1); -v(2),v(1),0];
end

% ---- Cross product ------------------------------------------------------
function c = cross3(a, b)
    c = [a(2)*b(3)-a(3)*b(2); a(3)*b(1)-a(1)*b(3); a(1)*b(2)-a(2)*b(1)];
end

% ---- Quaternion → DCM (body-to-NED) ------------------------------------
function R = quat2dcm(q)
    w=q(1); x=q(2); y=q(3); z=q(4);
    R = [w^2+x^2-y^2-z^2,  2*(x*y-w*z),      2*(x*z+w*y);
         2*(x*y+w*z),      w^2-x^2+y^2-z^2,  2*(y*z-w*x);
         2*(x*z-w*y),      2*(y*z+w*x),      w^2-x^2-y^2+z^2];
end

% ---- Euler → DCM -------------------------------------------------------
function R = euler2dcm(r, p, y)
    cr=cos(r); sr=sin(r); cp=cos(p); sp=sin(p); cy=cos(y); sy=sin(y);
    R = [cp*cy,          cp*sy,          -sp;
         sr*sp*cy-cr*sy, sr*sp*sy+cr*cy,  sr*cp;
         cr*sp*cy+sr*sy, cr*sp*sy-sr*cy,  cr*cp];
end

% ---- Euler → Quaternion -------------------------------------------------
function q = euler2quat(r, p, y)
    cr=cos(r/2); sr=sin(r/2);
    cp=cos(p/2); sp=sin(p/2);
    cy=cos(y/2); sy=sin(y/2);
    q = [cr*cp*cy + sr*sp*sy;
         sr*cp*cy - cr*sp*sy;
         cr*sp*cy + sr*cp*sy;
         cr*cp*sy - sr*sp*cy];
end

% ---- Quaternion → Euler -------------------------------------------------
function [r, p, y] = quat2euler(q)
    w=q(1); x=q(2); y_=q(3); z=q(4);
    r = atan2(2*(w*x + y_*z), 1 - 2*(x^2 + y_^2));
    p = asin(max(min(2*(w*y_ - z*x), 1), -1));
    y = atan2(2*(w*z + x*y_), 1 - 2*(y_^2 + z^2));
end

% ---- Quaternion conjugate -----------------------------------------------
function qc = qconj(q)
    qc = [q(1); -q(2); -q(3); -q(4)];
end

% ---- Quaternion multiplication ------------------------------------------
function qo = qmult(a, b)
    qo = [a(1)*b(1)-a(2)*b(2)-a(3)*b(3)-a(4)*b(4);
          a(1)*b(2)+a(2)*b(1)+a(3)*b(4)-a(4)*b(3);
          a(1)*b(3)-a(2)*b(4)+a(3)*b(1)+a(4)*b(2);
          a(1)*b(4)+a(2)*b(3)-a(3)*b(2)+a(4)*b(1)];
end

% ---- Exponential map: angle vector → quaternion -------------------------
function dq = expmap_quat(delta_ang)
    ang = norm(delta_ang);
    if ang > 1e-12
        ax = delta_ang / ang;
        dq = [cos(ang/2); ax * sin(ang/2)];
    else
        dq = [1; 0; 0; 0];
    end
end

% ---- Wrap angle to [-pi, pi] -------------------------------------------
function a = wrapToPi(a)
    a = mod(a + pi, 2*pi) - pi;
end

% ---- Apply bias inhibit to Kalman gain ----------------------------------
function K = apply_inhibit(K, gb_inh, ab_inh, IX_GB, IX_AB)
    for i = 1:3
        if gb_inh(i), K(IX_GB(i)) = 0; end
        if ab_inh(i), K(IX_AB(i)) = 0; end
    end
end

% ---- Update fail timer --------------------------------------------------
function tmr = update_fail_timer(tmr, is_failing, dt)
    if is_failing, tmr = tmr + dt; else, tmr = 0; end
end

% ---- 24-state fusion (apply Kalman gain to all states) ------------------
function [q,v,p,gb,ab,mI,mB,wv,tr] = ...
    fuse_state(q,v,p,gb,ab,mI,mB,wv,tr, K,inn, ...
               IA,IV,IP,IGB,IAB,IMI,IMB,IWV,ITR,GBL,ABL,MBL)

    % Attitude: axis-angle correction via exponential map
    da = K(IA) * inn;
    q = qmult(expmap_quat(da), q);
    q = q / norm(q);

    % Linear states with limits
    v  = max(min(v  + K(IV)*inn,  1000), -1000);
    p  = p  + K(IP)*inn;
    gb = max(min(gb + K(IGB)*inn, GBL),  -GBL);
    ab = max(min(ab + K(IAB)*inn, ABL),  -ABL);
    mI = max(min(mI + K(IMI)*inn, 1),    -1);
    mB = max(min(mB + K(IMB)*inn, MBL),  -MBL);
    wv = max(min(wv + K(IWV)*inn, 100),  -100);
    tr = max(min(tr + K(ITR)*inn, 10000),-10000);
end

% ---- Joseph form stabilized covariance update ---------------------------
function P = joseph_update(P, K, H, R, N)
    % P = (I - K*H)*P*(I - K*H)' + K*R*K'
    PH = P * H';
    for i = 1:N
        for j = 1:N
            P(i,j) = P(i,j) - K(i)*PH(j);
        end
    end
    PH = P * H';
    for i = 1:N
        for j = 1:i
            P(i,j) = P(i,j) - PH(i)*K(j) + K(i)*R*K(j);
            P(j,i) = P(i,j);
        end
    end
end

% ---- Delay buffer read (returns oldest or current if not full) ----------
function [da,dg,ddt, dp,dv,dgv, db,dbv, dm,dmv] = ...
    push_delay_buffer(acc,gyro,dt, gps_p,gps_v,gps_vld, ...
                      baro,baro_vld, mag,mag_vld, ...
                      ba,bg,bdt, bp,bv,bvld, bb,bbv,bm,bmv, ...
                      cnt, delay)
    if cnt < delay
        da=acc; dg=gyro; ddt=dt;
        dp=gps_p; dv=gps_v; dgv=gps_vld;
        db=baro; dbv=baro_vld;
        dm=mag; dmv=mag_vld;
    else
        da=ba(:,1); dg=bg(:,1); ddt=bdt(1);
        dp=bp(:,1); dv=bv(:,1); dgv=bvld(1);
        db=bb(1);   dbv=bbv(1);
        dm=bm(:,1); dmv=bmv(1);
    end
end

== matlab function UAM_Flight_control/Sensor/Subsystem1/GPS_Ref_Latch ==
  data: gps_lat input; ref_lat output; gps_lon input; gps_alt input; ref_lon output; ref_alt output
function [ref_lat, ref_lon, ref_alt] = GPS_Ref_Latch(gps_lat, gps_lon, gps_alt)
%#codegen
% Latch GPS reference at first valid sample, then hold it.

persistent initialized stored_lat stored_lon stored_alt

if isempty(initialized)
    initialized = false;
    stored_lat  = 0.0;
    stored_lon  = 0.0;
    stored_alt  = 0.0;
end

% validity (원하는 조건으로 조정 가능)
gps_valid = (gps_lat ~= 0) && (gps_lon ~= 0) && isfinite(gps_lat) && isfinite(gps_lon) && isfinite(gps_alt);

if ~initialized && gps_valid
    stored_lat  = gps_lat;
    stored_lon  = gps_lon;
    stored_alt  = gps_alt;
    initialized = true;
end

ref_lat = stored_lat;
ref_lon = stored_lon;
ref_alt = stored_alt;
end

== matlab function UAM_Flight_control/Sensor/Subsystem1/MATLAB Function6 ==
  data: gps_lat input; gps_valid output; gps_lon input; gps_alt input; gps_vel input; baro_alt input; mag input; baro_valid output; mag_valid output
function [gps_valid, baro_valid, mag_valid] = sensor_valid_check( ...
    gps_lat, gps_lon, gps_alt, gps_vel, ...
    baro_alt, ...
    mag)
%% SENSOR_VALID_CHECK  Sensor validity flags from raw values
%  GPS:  lat/lon이 유효 범위이고, 속도가 비정상이 아닌 경우
%  BARO: 고도값이 유효 범위인 경우
%  MAG:  자기장 크기가 지구 자기장 범위 내인 경우

%% ----- GPS VALIDITY -----
% 유효 위도: -90 ~ 90, 경도: -180 ~ 180, 둘 다 0이 아닌 실제 값
lat_ok  = (abs(gps_lat) >= 1e-6) && (abs(gps_lat) <= 90);
lon_ok  = (abs(gps_lon) >= 1e-6) && (abs(gps_lon) <= 180);
alt_ok  = (gps_alt > -1000) && (gps_alt < 100000);
vel_ok  = (norm(gps_vel) < 500);  % 500 m/s 이하
gps_valid = double(lat_ok && lon_ok && alt_ok && vel_ok);

%% ----- BARO VALIDITY -----
% 데이터 미수신 시 0이 들어오므로 abs >= 1 체크
% 기압 고도 유효 범위: -1000 ~ 100000 m
baro_valid = double((abs(baro_alt) >= 1) && (baro_alt > -1000) && (baro_alt < 100000));

%% ----- MAG VALIDITY -----
% 지구 자기장 크기: ~0.2 ~ 0.7 Gauss (20 ~ 70 uT)
mag_norm = norm(mag);
mag_valid = double((mag_norm > 0.1) && (mag_norm < 1.0));

end

== matlab function UAM_Flight_control/Controller/Manual/multicopter Controller/Horizontal Position Control1/MATLAB Function ==
  data: u input; y output; expo input
function y = expo_curve(u, expo)      

    y = sign(u) * (expo * abs(u)^3 + (1 - expo) * abs(u));   
    
end

== matlab function UAM_Flight_control/Controller/Manual/multicopter Controller/Horizontal Position Control1/MATLAB Function1 ==
  data: u input; y output; expo input
function y = expo_curve(u, expo)      

    y = sign(u) * (expo * abs(u)^3 + (1 - expo) * abs(u));   
    
end
